simulink model "pendoloSimulink"  (R2020a)
settings: Solver=VariableStepAuto  StartTime=0.0  StopTime=10.0  RelTol=1e-3
values from neighbouring files (symbols this model uses):
  g = @(uk1) uk1 -u(:,k-1) - h*feval(f,x(k),uk1)    [eulero_imp.m]    (also in eulero_implicito.m = @(uk1) uk1-u(k-1,:)-h*feval(f,x(k),uk1))
undefined symbols (not defined in the file or in its folder): l
settings Model: Creator=aless  LastModifiedBy=aless

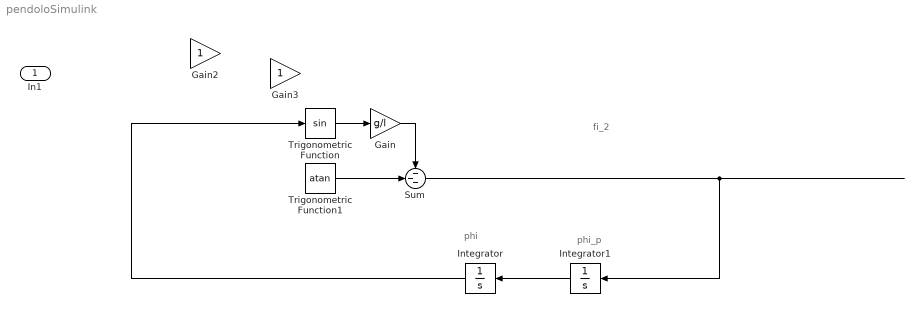
== system pendoloSimulink ==
  note: phi_p
  note: phi
  note: fi_2
  In1 : Inport
  Gain : Gain  Gain=g/l
  Gain2 : Gain
  Gain3 : Gain
  Integrator : Integrator
  Integrator1 : Integrator
  Sum : Sum  Inputs=---
  Trigonometric Function : Trigonometry
  Trigonometric Function1 : Trigonometry  Operator=atan
  wires:
  Trigonometric Function/1 -> Gain/1
  Sum/1 -> Integrator1/1
  Trigonometric Function1/1 -> Sum/2
  Integrator1/1 -> Integrator/1
  Integrator/1 -> Trigonometric Function/1
  Gain/1 -> Sum/1
